simulink model "Online_Ordering_System_Context_Diagram"  (R2024a)
settings: Solver=VariableStepAuto  StartTime=0.0  StopTime=10.0  RelTol=1e-3
settings Model: Creator=OdaNobuyuki  LastModifiedBy=chico

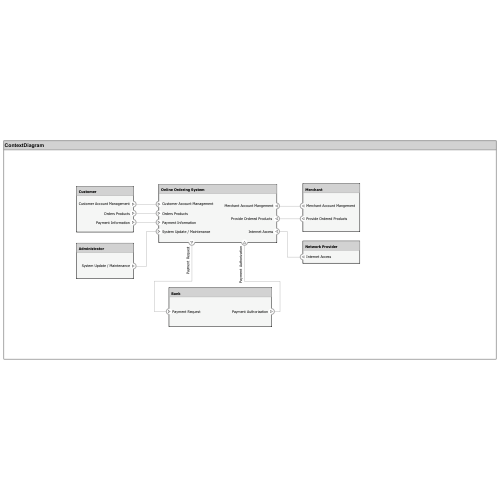
[thumbnail: Simulink's stored preview of the top-level diagram]
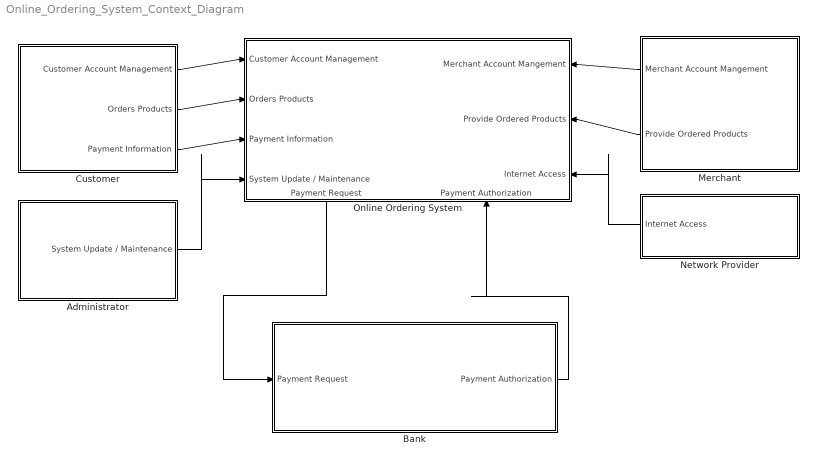
== system Online_Ordering_System_Context_Diagram ==
  Administrator : Subsystem
      settings: PortSchema="{\"entries\":[{\"content\":{\"headerSize\":26,\"margin\":15,\"minimumSpacing\":25,\"sides\":[{\"content\":{},\"type\":\"ConnectorPlacement.EquallySpacedRectSide\",\"uuid\":\"4bec0298-3227-49ac-a405-b42bbaee14f5\"},{\"content\":{\"connectorIds\":[\"Out1\"],\"side\":\"RIGHT\"},\"type\":\"ConnectorPlacement.EquallySpacedRectSide\",\"uuid\":\"1773ebbc-019c-4d02-a305-41c6e58a2de0\"},{\"content\":{\"side\":\"TOP\"},\"type\":\"ConnectorPlacement.EquallySpacedRectSide\",\"uuid\":\"4bd43937-d366-4309-882f-06c2ce5996af\"}]},\"type\":\"ConnectorPlacement.EquallySpacedConnector\",\"uuid\":\"7b1e0bc0-80f0-496e-8422-d8d80ac6cf10\"}],\"packageUris\":[\"http://schema.mathworks.com/mf0/Connector/R2020b\"],\"version\":\"1.0\"}"
  Bank : Subsystem
      settings: PortSchema="{\"entries\":[{\"content\":{\"headerSize\":26,\"margin\":15,\"minimumSpacing\":25,\"sides\":[{\"content\":{\"connectorIds\":[\"In1\"]},\"type\":\"ConnectorPlacement.EquallySpacedRectSide\",\"uuid\":\"4bec0298-3227-49ac-a405-b42bbaee14f5\"},{\"content\":{\"connectorIds\":[\"Out1\"],\"side\":\"RIGHT\"},\"type\":\"ConnectorPlacement.EquallySpacedRectSide\",\"uuid\":\"1773ebbc-019c-4d02-a305-41c6e58a2de0\"},{\"content\":{\"side\":\"TOP\"},\"type\":\"ConnectorPlacement.EquallySpacedRectSide\",\"uuid\":\"4bd43937-d366-4309-882f-06c2ce5996af\"}]},\"type\":\"ConnectorPlacement.EquallySpacedConnector\",\"uuid\":\"7b1e0bc0-80f0-496e-8422-d8d80ac6cf10\"}],\"packageUris\":[\"http://schema.mathworks.com/mf0/Connector/R2020b\"],\"version\":\"1.0\"}"
  Customer : Subsystem
      settings: PortSchema="{\"entries\":[{\"content\":{\"headerSize\":26,\"margin\":15,\"minimumSpacing\":25,\"sides\":[{\"content\":{},\"type\":\"ConnectorPlacement.EquallySpacedRectSide\",\"uuid\":\"4bec0298-3227-49ac-a405-b42bbaee14f5\"},{\"content\":{\"connectorIds\":[\"Out1\",\"Out2\",\"Out3\"],\"side\":\"RIGHT\"},\"type\":\"ConnectorPlacement.EquallySpacedRectSide\",\"uuid\":\"1773ebbc-019c-4d02-a305-41c6e58a2de0\"},{\"content\":{\"side\":\"TOP\"},\"type\":\"ConnectorPlacement.EquallySpacedRectSide\",\"uuid\":\"4bd43937-d366-4309-882f-06c2ce5996af\"}]},\"type\":\"ConnectorPlacement.EquallySpacedConnector\",\"uuid\":\"7b1e0bc0-80f0-496e-8422-d8d80ac6cf10\"}],\"packageUris\":[\"http://schema.mathworks.com/mf0/Connector/R2020b\"],\"version\":\"1.0\"}"
  Merchant : Subsystem
      settings: PortSchema="{\"entries\":[{\"content\":{\"headerSize\":26,\"margin\":15,\"minimumSpacing\":25,\"sides\":[{\"content\":{\"connectorIds\":[\"Out2\",\"Out1\"]},\"type\":\"ConnectorPlacement.EquallySpacedRectSide\",\"uuid\":\"4bec0298-3227-49ac-a405-b42bbaee14f5\"},{\"content\":{\"side\":\"RIGHT\"},\"type\":\"ConnectorPlacement.EquallySpacedRectSide\",\"uuid\":\"1773ebbc-019c-4d02-a305-41c6e58a2de0\"},{\"content\":{\"side\":\"TOP\"},\"type\":\"ConnectorPlacement.EquallySpacedRectSide\",\"uuid\":\"4bd43937-d366-4309-882f-06c2ce5996af\"}]},\"type\":\"ConnectorPlacement.EquallySpacedConnector\",\"uuid\":\"7b1e0bc0-80f0-496e-8422-d8d80ac6cf10\"}],\"packageUris\":[\"http://schema.mathworks.com/mf0/Connector/R2020b\"],\"version\":\"1.0\"}"
  Network Provider : Subsystem
      settings: PortSchema="{\"entries\":[{\"content\":{\"headerSize\":26,\"margin\":15,\"minimumSpacing\":25,\"sides\":[{\"content\":{\"connectorIds\":[\"Out1\"]},\"type\":\"ConnectorPlacement.EquallySpacedRectSide\",\"uuid\":\"4bec0298-3227-49ac-a405-b42bbaee14f5\"},{\"content\":{\"side\":\"RIGHT\"},\"type\":\"ConnectorPlacement.EquallySpacedRectSide\",\"uuid\":\"1773ebbc-019c-4d02-a305-41c6e58a2de0\"},{\"content\":{\"side\":\"TOP\"},\"type\":\"ConnectorPlacement.EquallySpacedRectSide\",\"uuid\":\"4bd43937-d366-4309-882f-06c2ce5996af\"}]},\"type\":\"ConnectorPlacement.EquallySpacedConnector\",\"uuid\":\"7b1e0bc0-80f0-496e-8422-d8d80ac6cf10\"}],\"packageUris\":[\"http://schema.mathworks.com/mf0/Connector/R2020b\"],\"version\":\"1.0\"}"
  Online Ordering System : Subsystem
      settings: PortSchema="{\"entries\":[{\"content\":{\"headerSize\":26,\"margin\":15,\"minimumSpacing\":25,\"sides\":[{\"content\":{\"connectorIds\":[\"In6\",\"In2\",\"In3\",\"In7\"]},\"type\":\"ConnectorPlacement.EquallySpacedRectSide\",\"uuid\":\"4bec0298-3227-49ac-a405-b42bbaee14f5\"},{\"content\":{\"connectorIds\":[\"In1\",\"In4\",\"In5\"],\"side\":\"RIGHT\"},\"type\":\"ConnectorPlacement.EquallySpacedRectSide\",\"uuid\":\"1773ebbc-019c-4d02-a305-41c6e58a2de0\"},{\"content\":{\"side\":\"TOP\"},\"type\":\"ConnectorPlacement.EquallySpacedRectSide\",\"uuid\":\"4bd43937-d366-4309-882f-06c2ce5996af\"},{\"content\":{\"connectorIds\":[\"Out1\",\"In8\"],\"side\":\"BOTTOM\"},\"type\":\"ConnectorPlacement.EquallySpacedRectSide\",\"uuid\":\"7e5ccc30-c91d-47eb-83c6-f8eaa47ffc39\"}]},\"type\":\"ConnectorPlacement.EquallySpacedConnector\",\"uuid\":\"7b1e0bc0-80f0-496e-8422-d8d80ac6cf10\"}],\"packageUris\":[\"http://schema.mathworks.com/mf0/Connector/R2020b\"],\"version\":\"1.0\"}"
  wires:
  Merchant/1("Provide Ordered Products ") -> Online Ordering System/4("Provide Ordered Products ")
  Merchant/2(Merchant Account Mangement) -> Online Ordering System/1(Merchant Account Mangement)
  Customer/1(Customer Account Management) -> Online Ordering System/6(Customer Account Management)
  Network Provider/1(Internet Access) -> Online Ordering System/5(Internet Access)
  Customer/3(Payment Information) -> Online Ordering System/3(Payment Information)
  Customer/2(Orders Products) -> Online Ordering System/2(Orders Products)
  Administrator/1(System Update / Maintenance) -> Online Ordering System/7(System Update / Maintenance)
  Online Ordering System/1(Payment Request) -> Bank/1(Payment Request)
  Bank/1(Payment Authorization) -> Online Ordering System/8(Payment Authorization)

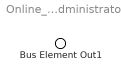
== system Online_Ordering_System_Context_Diagram/Administrator ==
  Bus Element Out1 : Outport  PortName=System Update / Maintenance

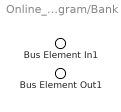
== system Online_Ordering_System_Context_Diagram/Bank ==
  Bus Element In1 : Inport  PortName=Payment Request
  Bus Element Out1 : Outport  PortName=Payment Authorization

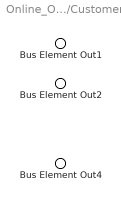
== system Online_Ordering_System_Context_Diagram/Customer ==
  Bus Element Out1 : Outport  PortName=Customer Account Management
  Bus Element Out2 : Outport  Port=2  PortName=Orders Products
  Bus Element Out4 : Outport  Port=3  PortName=Payment Information

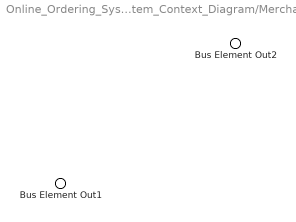
== system Online_Ordering_System_Context_Diagram/Merchant ==
  Bus Element Out2 : Outport  PortName=Provide Ordered Products
  Bus Element Out1 : Outport  Port=2  PortName=Merchant Account Mangement

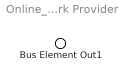
== system Online_Ordering_System_Context_Diagram/Network Provider ==
  Bus Element Out1 : Outport  PortName=Internet Access

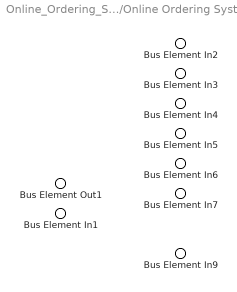
== system Online_Ordering_System_Context_Diagram/Online Ordering System ==
  Bus Element In4 : Inport  PortName=Merchant Account Mangement
  Bus Element In7 : Inport  Port=2  PortName=Orders Products
  Bus Element In9 : Inport  Port=3  PortName=Payment Information
  Bus Element In6 : Inport  Port=4  PortName=Provide Ordered Products
  Bus Element In5 : Inport  Port=5  PortName=Internet Access
  Bus Element In2 : Inport  Port=6  PortName=Customer Account Management
  Bus Element In3 : Inport  Port=7  PortName=System Update / Maintenance
  Bus Element In1 : Inport  Port=8  PortName=Payment Authorization
  Bus Element Out1 : Outport  PortName=Payment Request
